simulink model "battery_dis"  (R2019b)
settings: Solver=VariableStepAuto  StartTime=0.0  StopTime=tsimulation  RelTol=1e-3
values from neighbouring files (symbols this model uses):
  C = Cbat*Nbp*3600    (= 37440)    [demoEPS.m]    (also in demoEPS_R2019a.m; demoEPS_v1.m; demoEPS_v1a.m; demoEPS_v1test.m)
  DOD_0 = 0    [demoEPS.m]    (also in demoEPS_R2019a.m; demoEPS_v1.m; demoEPS_v1a.m; demoEPS_v1test.m)
  eff_i1 = 0.9    [demoEPS.m]    (also in demoEPS_R2019a.m; demoEPS_v1.m; demoEPS_v1a.m; demoEPS_v1test.m)
  iLoad = 2    [testsim.m]
  Nbs = math.ceil(Vbusmin/Vbatmin)    [calc_mass_EPS.m]    (also in demoEPS.m = 4; demoEPS_R2019a.m = 4; demoEPS_v1.m = 4; demoEPS_v1a.m = 4)
  Pload = 50    [testsim.m]
libraries: simulink x2
settings Model: Creator=Ricardo  LastModifiedBy=Ricardo

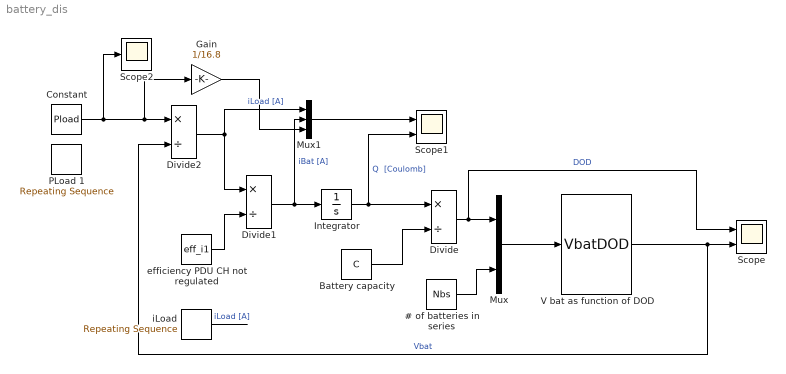
== system battery_dis ==
  # of batteries in series : Constant  Value=Nbs
  Battery capacity : Constant  Value=C
  Constant : Constant  Value=Pload
  Divide : Product  Inputs=*/
  Divide1 : Product  Inputs=*/
  Divide2 : Product  Inputs=*/
  Gain : Gain  Gain=1/16.8
  Integrator : Integrator  InitialCondition=DOD_0
  Mux : Mux  Inputs=2
  Mux1 : Mux  Inputs=3
  PLoad 1 : simulink/Sources/Repeating Sequence  rep_seq_t=[0 300 300.1 350]  rep_seq_y=[Pload Pload 0 0]
  Scope : Scope  NumInputPorts=2
  Scope1 : Scope  NumInputPorts=2
  Scope2 : Scope
  V bat as function of DOD : MATLABFcn  MATLABFcn=VbatDOD
  efficiency PDU CH not regulated : Constant  Value=eff_i1
  iLoad : simulink/Sources/Repeating Sequence  rep_seq_t=[0 5 5.1 10]  rep_seq_y=[iLoad iLoad 0 0]
  wires:
  Mux/1 -> V bat as function of DOD/1
  # of batteries in series/1 -> Mux/2
  V bat as function of DOD/1 -> Divide2/2, Scope/2  "Vbat"
  Divide/1 -> Scope/1, Mux/1  "DOD"
  Divide1/1 -> Mux1/2, Integrator/1  "iBat [A]"
  Integrator/1 -> Scope1/2, Divide/1  "Q  [Coulomb]"
  Battery capacity/1 -> Divide/2
  iLoad/1 -> ?  "iLoad [A]"
  efficiency PDU CH not regulated/1 -> Divide1/2
  Divide2/1 -> Mux1/1, Divide1/1  "iLoad [A]"
  Mux1/1 -> Scope1/1
  Gain/1 -> Mux1/3
  Constant/1 -> Scope2/1, Gain/1, Divide2/1
